simulink model "Thruster_Example_rw"  (R2024b)
settings: Solver=ode4  StartTime=0.0  StopTime=2000  FixedStep=0.01  RelTol=1e-3
undefined symbols (not defined in the file): Cube_L, dt, F_vec, Iws, M_rw, m_tot, norm_Ib, Omega1_init, Omega2_init, Omega3_init, Omega4_init, qb0, rad2rpm, RCS_F, RCS_F_vec, RCS_Pos, RCS_pos, RCS_PWM_Freq, RCS_Sampling_time, RCS_THR_vec, REL_TS_POS_I_0, REL_TS_VEL_I_0, RW_As, RW_Max_Speed, RW_Omegad_max, sat, SC_Ib, SC_state0, SS_Total_Mass, TC_Kepler, THR_dt, THR_Force, THR_freq, THR_Pos, TS_Ib, TS_qb0, TS_state0, TS_wb0, wb0, X, Y, Z
libraries: sm_lib x348, nesl_utility x236, simulink_extras x115, sharedtransform x64, aerolibutil x38, simulink x28, sharedutil x13
(part 15 of 16)

== matlab function Thruster_Example_rw/Reaction_Wheel_Simple1/quaternion to Euler angle 1 ==
  data: angle output; q input
function angle = quat2eulang(q)
% ZYX 회전 가정

% q0 = q(1); q1 = q(2); q2 = q(3); q3 = q(4);
% 
% yaw = atan2(2*(q1*q2 + q0*q3), q0^2+q1^2-q2^2-q3^2);
% 
% s = 2*(q0*q2 - q3*q1);
% s = max(-1, min(1, s));      % clamp
% pitch = asin(s);
% 
% roll = atan2(2*(q2*q3 + q0*q1), q0^2-q1^2-q2^2+q3^2);



% % 'ZYX' 회전에서 DCM을 Body-frame -> 관성좌표계 으로 정의할 때, 각을 구하는 상황.
% % /                cos(psi) cos(theta),                              cos(theta) sin(psi),                   -sin(theta)     \
% % |                                                                                                                         |
% % | cos(psi) sin(phi) sin(theta) - cos(phi) sin(psi), cos(phi) cos(psi) + sin(phi) sin(psi) sin(theta), cos(theta) sin(phi) |
% % |                                                                                                                         |
% % \ sin(phi) sin(psi) + cos(phi) cos(psi) sin(theta), cos(phi) sin(psi) sin(theta) - cos(psi) sin(phi), cos(phi) cos(theta) /
R = quat2DCM(q);
yaw   = atan2(R(1,2), R(1,1));
pitch = -asin(R(1,3));
roll  = atan2(R(2,3), R(3,3));



% angle = [roll, pitch, yaw]';
angle = [yaw, pitch, roll]'; %MATLAB 에서는 [roll, pitch, yaw] 가 아닌 [yaw, pitch, roll] 순으로 값을 반환한다.
% 실제 도움말을 보면, 반환각 벡터에 대해 "Ψ is R1, Θ is R2, and Φ is R3." 으로 나와있는 것을 볼 수 있다.



function R = quat2DCM(q)

q0 = q(1); q1 = q(2); q2 = q(3); q3 = q(4);

%% DCM을 관성좌표계 -> Body-frame 으로 정의할 때의 행렬 
% R = [2*(q0^2 + q1^2)-1, 2*(q1*q2 - q0*q3),2*(q1*q3 + q2*q0);
%      2*(q1*q2 + q0*q3), 2*(q0^2 + q2^2)-1, 2*(q2*q3 - q1*q0);
%      2*(q1*q3 - q2*q0), 2*(q2*q3 + q1*q0), 2*(q0^2 + q3^2)-1];

%% DCM을 Body-frame -> 관성좌표계 으로 정의할 때의 행렬 
R = [q0^2+q1^2-q2^2-q3^2, 2*(q1*q2 + q0*q3), 2*(q1*q3 - q2*q0);
     2*(q1*q2 - q0*q3), q0^2-q1^2+q2^2-q3^2, 2*(q2*q3 + q1*q0);
     2*(q1*q3 + q2*q0), 2*(q2*q3 - q1*q0), q0^2-q1^2-q2^2+q3^2];

end

end

== matlab function Thruster_Example_rw/Prac1/RCS_Position&Attitude_Controller ==
  settings: updateMethod=DISCRETE
  data: r_rel input; v_rel input; r_ref input; v_ref input; a_ref input; q input; q_err input; w_err input; wb input; F_cmd_B output; tau_cmd_B output; m_sc input; Ib input; Kp_pos input; Kd_pos input; Kp_att input; Kd_att input; r_err output; v_err output; q output; q_err_vec output; w_err output; a_cmd output
function [F_cmd_B, tau_cmd_B, r_err, v_err, q, q_err_vec, w_err, a_cmd] = ...
    relative_position_los_controller( ...
    r_rel, v_rel, ...          % [3x1] relative position/velocity
    r_ref, v_ref, a_ref, ...   % [3x1] desired relative pos/vel/acc
    q, q_err, w_err, wb, m_sc, Ib, Kp_pos, Kd_pos, Kp_att, Kd_att)
%#codegen
%
% q, q_los_ref : scalar-first quaternion [qw qx qy qz]'
%                body -> reference
% r_rel, r_ref, v_rel, v_ref, a_ref : reference frame 기준
%
% 출력:
% F_cmd_B   : [3x1] body frame force command
% tau_cmd_B : [3x1] body frame torque command

F_cmd_B   = zeros(3,1);
tau_cmd_B = zeros(3,1);
r_err     = zeros(3,1);
v_err     = zeros(3,1);
q_err_vec = zeros(3,1);
% w_err     = zeros(3,1);
a_cmd     = zeros(3,1);

%% 1) Relative position controller
r_err = r_ref - r_rel;
v_err = v_ref - v_rel;

a_cmd = a_ref + Kp_pos * r_err + Kd_pos * v_err;
F_cmd_R = m_sc * a_cmd;

%% 2) Reference frame -> body frame
% q : body -> reference
% therefore F_B = C_BR' * F_R
C_BR   = quat_to_dcm_sf(q);
F_cmd_B = C_BR' * F_cmd_R;

%% 3) LOS attitude controller

% shortest path
% if q_err(1) < 0
%     q_err = -q_err;
% end

q_err_vec = q_err(2:4);

tau_cmd_B = Kp_att * q_err_vec + Kd_att * w_err + cross(wb, Ib*wb);
end


function q_out = quat_mul_sf(a, b)
% scalar-first quaternion multiplication
q_out = [ a(1)*b(1) - a(2)*b(2) - a(3)*b(3) - a(4)*b(4);
    a(1)*b(2) + a(2)*b(1) + a(3)*b(4) - a(4)*b(3);
    a(1)*b(3) - a(2)*b(4) + a(3)*b(1) + a(4)*b(2);
    a(1)*b(4) + a(2)*b(3) - a(3)*b(2) + a(4)*b(1) ];
end


function C = quat_to_dcm_sf(q)
% scalar-first quaternion, body -> reference
q = q / (sqrt(sum(q.^2)) + 1e-12);

qw = q(1);
qx = q(2);
qy = q(3);
qz = q(4);

C = [1-2*(qy*qy+qz*qz),   2*(qx*qy-qw*qz),   2*(qx*qz+qw*qy);
    2*(qx*qy+qw*qz),     1-2*(qx*qx+qz*qz), 2*(qy*qz-qw*qx);
    2*(qx*qz-qw*qy),     2*(qy*qz+qw*qx),   1-2*(qx*qx+qy*qy)];
end

== matlab function Thruster_Example_rw/Reaction_Wheel_Simple1/deriviation of quaternion1 ==
  data: w input; q_prime output; q input
function q_prime = fcn(w,q)

F_q = (1/2)*[0 -w(1) -w(2) -w(3);
       w(1) 0 w(3) -w(2);
       w(2) -w(3) 0 w(1);
       w(3) w(2) -w(1) 0];

q_prime = F_q*q;

== matlab function Thruster_Example_rw/Prac1/RCS_Relative_Position_Control_Allocation2 ==
  settings: updateMethod=DISCRETE
  data: F_cmd input; tau_cmd input; RCS_pos input; RCS_F_vec input; Tmax input; duty output; F_est output; tau_est output; F_err output; tau_err output; sat_ratio output; wF input; wT input
function [duty, F_est, tau_est, F_err, tau_err, sat_ratio] = ...
    rcs_force_torque_allocator(F_cmd, tau_cmd, RCS_pos, RCS_F_vec, Tmax, wF, wT)
%#codegen
%
% F_cmd      : [3x1] commanded force in body frame [N]
% tau_cmd    : [3x1] commanded torque in body frame [N*m]
% RCS_pos    : [3xN] thruster positions in body frame [m]
% RCS_F_vec  : [3xN] thruster direction vectors
% Tmax       : scalar, max thrust of one thruster [N]
% wF         : scalar, force tracking weight
% wT         : scalar, torque tracking weight
%
% duty       : [N x 1], 0~1
% F_est      : [3x1], achieved force [N]
% tau_est    : [3x1], achieved torque [N*m]
% F_err      : [3x1], force error [N]
% tau_err    : [3x1], torque error [N*m]
% sat_ratio  : saturated thruster ratio

    N = size(RCS_pos, 2);

    duty      = zeros(N,1);
    F_est     = zeros(3,1);
    tau_est   = zeros(3,1);
    F_err     = zeros(3,1);
    tau_err   = zeros(3,1);
    sat_ratio = 0;

    Fmat = zeros(3, N);
    Tmat = zeros(3, N);

    for i = 1:N
        dir_i = RCS_F_vec(:,i);
        nrm   = sqrt(sum(dir_i.^2));

        if nrm > 1e-12
            dir_i = dir_i / nrm;
        else
            dir_i = [0;0;0];
        end

        Fi = Tmax * dir_i;
        Ti = cross3(RCS_pos(:,i), Fi);

        Fmat(:,i) = Fi;
        Tmat(:,i) = Ti;
    end

    % Solve:
    % min || wF*(Fmat*u - F_cmd) ||^2 + || wT*(Tmat*u - tau_cmd) ||^2
    % s.t. 0 <= u <= 1

    A = [wF * Fmat;
         wT * Tmat];

    b = [wF * F_cmd;
         wT * tau_cmd];

    H = A' * A + 1e-8 * eye(N);
    g = A' * b;

    alpha = 1.0 / (trace(H) + 1e-9);
    u = zeros(N,1);

    for k = 1:150
        grad = H * u - g;
        u    = u - alpha * grad;

        for j = 1:N
            if u(j) < 0
                u(j) = 0;
            elseif u(j) > 1
                u(j) = 1;
            end
        end
    end

    duty    = u;
    F_est   = Fmat * duty;
    tau_est = Tmat * duty;

    F_err   = F_cmd   - F_est;
    tau_err = tau_cmd - tau_est;

    sat_ratio = sum(duty > 0.999) / N;
end


function c = cross3(a, b)
    c = [ a(2)*b(3) - a(3)*b(2);
          a(3)*b(1) - a(1)*b(3);
          a(1)*b(2) - a(2)*b(1) ];
end

== matlab function Thruster_Example_rw/Reaction_Wheel_3axis/deriviation of quaternion2 ==
  data: w input; q_prime output; q input
function q_prime = fcn(w,q)

F_q = (1/2)*[0 -w(1) -w(2) -w(3);
       w(1) 0 w(3) -w(2);
       w(2) -w(3) 0 w(1);
       w(3) w(2) -w(1) 0];

q_prime = F_q*q;

== matlab function Thruster_Example_rw/Prac1/SC 6-DOF Dynamics ==
  data: w input; x input; Ib input; m_tot input; Iws input; As input; Omega input; Omegad input; RCS_mea input; RCS_pos input; RCS_vec input; wd output; R_Ib input; T_ext input; F_ext input; xd output
function [wd, xd]  = eq_propagate(w, x, Ib, m_tot, ...
                                   Iws, As, Omega, Omegad, ...
                                   RCS_mea, RCS_pos, RCS_vec, R_Ib, ...
                                   T_ext, F_ext)
% % 
% 출력 1: 위성 동체 좌표계 각가속도
% 출력 2: 관성좌표계 선가속도

RW_h = As*Iws*Omega;
RW_hd = As*Iws*Omegad;
% 
% % % 
% N = 16;
% RCS_f = zeros(3,N);
% RCS_t = zeros(3,N);
% 
% for i = 1:N
%     r_i = RCS_pos(:,i);   % position of thruster i
%     d_i = RCS_vec(:,i);   % thrust direction of thruster i
% 
%     % force contribution
%     RCS_f(:,i) = d_i;
% 
%     % torque contribution
%     RCS_t(:,i) = cross(r_i, d_i);
% end
% RCS_f_total = RCS_f * RCS_mea;  % [3x1]
% RCS_t_total = RCS_t * RCS_mea;  % [3x1]


%% Rotational Motion
wd = [0 0 0]';
wd = inv(Ib)*(T_ext - RW_hd - cross(w, Ib*w + RW_h));

%% Translational Motion

% F_I = R_Ib * RCS_f_total;
F_I = [0 0 0]';

u  = 3.9860064e+14; % earth gravitional parameter
Re = 6378137;      % earth radius [m]

xd = zeros(size(x));

v1_i = x(4); % x1 = dx/dt
v2_i = x(5); % y1 = dy/dt
v3_i = x(6); % z1 = dz/dt
p1_i = x(1); % x
p2_i = x(2); % y
p3_i = x(3); % z

r=sqrt(p1_i^2+p2_i^2+p3_i^2);

% % %   Keplar Motion Equatnion
% % %  => r_dd + u/(r^3)r_ = 0 => r_dd = -u/(r^3)r_
xd(1) = v1_i;
xd(2) = v2_i;
xd(3) = v3_i;
xd(4) = -u*p1_i/(r^3) + F_I(1)/m_tot + F_ext(1)/m_tot;
xd(5) = -u*p2_i/(r^3) + F_I(2)/m_tot + F_ext(2)/m_tot;
xd(6) = -u*p3_i/(r^3) + F_I(3)/m_tot + F_ext(3)/m_tot;

end

== matlab function Thruster_Example_rw/Reaction_Wheel_3axis/quaternion to Euler angle 1 ==
  data: angle output; q input
function angle = quat2eulang(q)
% ZYX 회전 가정

% q0 = q(1); q1 = q(2); q2 = q(3); q3 = q(4);
% 
% yaw = atan2(2*(q1*q2 + q0*q3), q0^2+q1^2-q2^2-q3^2);
% 
% s = 2*(q0*q2 - q3*q1);
% s = max(-1, min(1, s));      % clamp
% pitch = asin(s);
% 
% roll = atan2(2*(q2*q3 + q0*q1), q0^2-q1^2-q2^2+q3^2);



% % 'ZYX' 회전에서 DCM을 Body-frame -> 관성좌표계 으로 정의할 때, 각을 구하는 상황.
% % /                cos(psi) cos(theta),                              cos(theta) sin(psi),                   -sin(theta)     \
% % |                                                                                                                         |
% % | cos(psi) sin(phi) sin(theta) - cos(phi) sin(psi), cos(phi) cos(psi) + sin(phi) sin(psi) sin(theta), cos(theta) sin(phi) |
% % |                                                                                                                         |
% % \ sin(phi) sin(psi) + cos(phi) cos(psi) sin(theta), cos(phi) sin(psi) sin(theta) - cos(psi) sin(phi), cos(phi) cos(theta) /
R = quat2DCM(q);
yaw   = atan2(R(1,2), R(1,1));
pitch = -asin(R(1,3));
roll  = atan2(R(2,3), R(3,3));



% angle = [roll, pitch, yaw]';
angle = [yaw, pitch, roll]'; %MATLAB 에서는 [roll, pitch, yaw] 가 아닌 [yaw, pitch, roll] 순으로 값을 반환한다.
% 실제 도움말을 보면, 반환각 벡터에 대해 "Ψ is R1, Θ is R2, and Φ is R3." 으로 나와있는 것을 볼 수 있다.



function R = quat2DCM(q)

q0 = q(1); q1 = q(2); q2 = q(3); q3 = q(4);

%% DCM을 관성좌표계 -> Body-frame 으로 정의할 때의 행렬 
% R = [2*(q0^2 + q1^2)-1, 2*(q1*q2 - q0*q3),2*(q1*q3 + q2*q0);
%      2*(q1*q2 + q0*q3), 2*(q0^2 + q2^2)-1, 2*(q2*q3 - q1*q0);
%      2*(q1*q3 - q2*q0), 2*(q2*q3 + q1*q0), 2*(q0^2 + q3^2)-1];

%% DCM을 Body-frame -> 관성좌표계 으로 정의할 때의 행렬 
R = [q0^2+q1^2-q2^2-q3^2, 2*(q1*q2 + q0*q3), 2*(q1*q3 - q2*q0);
     2*(q1*q2 - q0*q3), q0^2-q1^2+q2^2-q3^2, 2*(q2*q3 + q1*q0);
     2*(q1*q3 + q2*q0), 2*(q2*q3 - q1*q0), q0^2-q1^2-q2^2+q3^2];

end

end

== matlab function Thruster_Example_rw/Reaction_Wheel_Simple3/deriviation of quaternion2 ==
  data: w input; q_prime output; q input
function q_prime = fcn(w,q)

F_q = (1/2)*[0 -w(1) -w(2) -w(3);
       w(1) 0 w(3) -w(2);
       w(2) -w(3) 0 w(1);
       w(3) w(2) -w(1) 0];

q_prime = F_q*q;

== matlab function Thruster_Example_rw/Reaction_Wheel_Simple3/rigid body2 ==
  data: Wheel_MOI input; Ib input; t_ext input; omega_prime output; omega input; omega_rw input; omega_rw_prime input
function omega_prime = fcn(Wheel_MOI, Ib, t_ext, omega,omega_rw,omega_rw_prime)
% L = [0.3 0.3 0.3]'; %Length([m]) of cube 
% M = 10; %Mass([kg]) of cube
% MOI([kg*m^2]) of cube
% I = [ 1/12*M*(L(2)^2+L(3)^2) 0 0;
%       0 1/12*M*(L(1)^2+L(3)^2) 0;
%       0 0 1/12*M*(L(1)^2+L(2)^2)];

% R=0.015; % Radius([m]) of cylinder(Reaction wheel)
% M_rw=0.01; % Mass([kg]) of cylinder(Reaction wheel)
% L_rw=0.01; % Length([m]) of cylinder(Reaction wheel)

% MOI([kg*m^2]) of cylinder(Reaction wheel)
% I_rw=[1/4*M_rw*R^2+1/12*M_rw*L_rw^2 0 0;
%     0 1/4*M_rw*R^2+1/12*M_rw*L_rw^2 0;
%     0 0 1/2*M_rw*R^2];
% Ib=I;

I_rw3 = Wheel_MOI(3,3);
I_rw = diag([0 0 I_rw3]);

As1 = [0 0 0]';
As2 = [0 0 0]';
As3 = [0 -sind(45) cosd(45)]';

As = [As1, As2, As3];

omega_prime = inv(Ib)*(t_ext - As*I_rw*omega_rw_prime - cross(omega, (Ib*omega) + As*I_rw*omega_rw));

end

== matlab function Thruster_Example_rw/Reaction_Wheel_3axis/rigid body2 ==
  data: Ib input; t_ext input; omega_prime output; omega input; omega_rw input; omega_rw_prime input; R_rw input; L_rw input; M_rw input
function omega_prime = fcn(Ib, t_ext, omega,omega_rw,omega_rw_prime, R_rw, L_rw, M_rw)
L = [0.3 0.3 0.3]'; %Length([m]) of cube 
M = 10; %Mass([kg]) of cube
% MOI([kg*m^2]) of cube
I = [ 1/12*M*(L(2)^2+L(3)^2) 0 0;
      0 1/12*M*(L(1)^2+L(3)^2) 0;
      0 0 1/12*M*(L(1)^2+L(2)^2)];

% R=0.015; % Radius([m]) of cylinder(Reaction wheel)
% L_rw=0.01; % Length([m]) of cylinder(Reaction wheel)
% M_rw=0.01; % Mass([kg]) of cylinder(Reaction wheel)
R=R_rw;


% MOI([kg*m^2]) of cylinder(Reaction wheel)
I_rw=[1/4*M_rw*R^2+1/12*M_rw*L_rw^2 0 0;
    0 1/4*M_rw*R^2+1/12*M_rw*L_rw^2 0;
    0 0 1/2*M_rw*R^2];

% Ib=I;


omega_prime = inv(Ib)*(t_ext - I_rw*omega_rw_prime - cross(omega, (Ib*omega) + I_rw*omega_rw));

end

== matlab function Thruster_Example_rw/Reaction_Wheel_Simple2/deriviation of quaternion2 ==
  data: w input; q_prime output; q input
function q_prime = fcn(w,q)

F_q = (1/2)*[0 -w(1) -w(2) -w(3);
       w(1) 0 w(3) -w(2);
       w(2) -w(3) 0 w(1);
       w(3) w(2) -w(1) 0];

q_prime = F_q*q;

== matlab function Thruster_Example_rw/Single_Reaction_Wheel_PD_Control/deriviation of quaternion2 ==
  data: w input; q_prime output; q input
function q_prime = fcn(w,q)

F_q = (1/2)*[0 -w(1) -w(2) -w(3);
       w(1) 0 w(3) -w(2);
       w(2) -w(3) 0 w(1);
       w(3) w(2) -w(1) 0];

q_prime = F_q*q;

== matlab function Thruster_Example_rw/Single_Reaction_Wheel_PD_Control/rigid body2 ==
  data: Wheel_MOI input; Ib input; t_ext input; omega_prime output; omega input; omega_rw input; omega_rw_prime input
function omega_prime = fcn(Wheel_MOI, Ib, t_ext, omega,omega_rw,omega_rw_prime)
% L = [0.3 0.3 0.3]'; %Length([m]) of cube 
% M = 10; %Mass([kg]) of cube
% MOI([kg*m^2]) of cube
% I = [ 1/12*M*(L(2)^2+L(3)^2) 0 0;
%       0 1/12*M*(L(1)^2+L(3)^2) 0;
%       0 0 1/12*M*(L(1)^2+L(2)^2)];

% R=0.015; % Radius([m]) of cylinder(Reaction wheel)
% M_rw=0.01; % Mass([kg]) of cylinder(Reaction wheel)
% L_rw=0.01; % Length([m]) of cylinder(Reaction wheel)

% MOI([kg*m^2]) of cylinder(Reaction wheel)
% I_rw=[1/4*M_rw*R^2+1/12*M_rw*L_rw^2 0 0;
%     0 1/4*M_rw*R^2+1/12*M_rw*L_rw^2 0;
%     0 0 1/2*M_rw*R^2];
% Ib=I;

I_rw3 = Wheel_MOI(3,3);
I_rw = diag([0 0 I_rw3]);

As1 = [0 0 0]';
As2 = [0 0 0]';
As3 = [0 -sind(45) cosd(45)]';

As = [As1, As2, As3];

omega_prime = inv(Ib)*(t_ext - As*I_rw*omega_rw_prime - cross(omega, (Ib*omega) + As*I_rw*omega_rw));

end

== matlab function Thruster_Example_rw/Single_Reaction_Wheel_PD_Control/rigid body1 ==
  data: yaw_err input; w_z_err input; u_cntl output
function u_cntl = fcn(yaw_err, w_z_err)

K1 = 0.0;
K2 = 100000.0;

u_cntl = K1*yaw_err + K2*w_z_err;


end

== matlab function Thruster_Example_rw/Reaction_Wheel_another_Position/deriviation of quaternion2 ==
  data: w input; q_prime output; q input
function q_prime = fcn(w,q)

F_q = (1/2)*[0 -w(1) -w(2) -w(3);
       w(1) 0 w(3) -w(2);
       w(2) -w(3) 0 w(1);
       w(3) w(2) -w(1) 0];

q_prime = F_q*q;

== matlab function Thruster_Example_rw/Reaction_Wheel_Simple2/rigid body2 ==
  data: Wheel_MOI input; Ib input; t_ext input; omega_prime output; omega input; omega_rw input; omega_rw_prime input
function omega_prime = fcn(Wheel_MOI, Ib, t_ext, omega,omega_rw,omega_rw_prime)
% L = [0.3 0.3 0.3]'; %Length([m]) of cube 
% M = 10; %Mass([kg]) of cube
% MOI([kg*m^2]) of cube
% I = [ 1/12*M*(L(2)^2+L(3)^2) 0 0;
%       0 1/12*M*(L(1)^2+L(3)^2) 0;
%       0 0 1/12*M*(L(1)^2+L(2)^2)];

% R=0.015; % Radius([m]) of cylinder(Reaction wheel)
% M_rw=0.01; % Mass([kg]) of cylinder(Reaction wheel)
% L_rw=0.01; % Length([m]) of cylinder(Reaction wheel)

% MOI([kg*m^2]) of cylinder(Reaction wheel)
% I_rw=[1/4*M_rw*R^2+1/12*M_rw*L_rw^2 0 0;
%     0 1/4*M_rw*R^2+1/12*M_rw*L_rw^2 0;
%     0 0 1/2*M_rw*R^2];
% Ib=I;

I_rw1 = Wheel_MOI(3,3);
I_rw = diag([I_rw1 I_rw1 I_rw1]);

omega_prime = inv(Ib)*(t_ext - I_rw*omega_rw_prime - cross(omega, (Ib*omega) + I_rw*omega_rw));

end

== matlab function Thruster_Example_rw/Reaction_Wheel_another_Position/rigid body2 ==
  data: Wheel_MOI input; Ib input; t_ext input; omega_prime output; omega input; omega_rw input; omega_rw_prime input
function omega_prime = fcn(Wheel_MOI, Ib, t_ext, omega,omega_rw,omega_rw_prime)

% Ib = diag([0.15, 0.15, 0.15]);
I_rw3 = Wheel_MOI(3,3);
% I_rw3 = 0.001125;

I_rw = diag([0 0 I_rw3]);

As1 = [0 0 0]';
As2 = [0 0 0]';
% As3 = [0 -sind(45) cosd(45)]';
As3 = [0 0 1]';

As = [As1, As2, As3];

omega_prime = inv(Ib)*(t_ext - As*I_rw*omega_rw_prime - cross(omega, (Ib*omega) + As*I_rw*omega_rw));

end

== matlab function Thruster_Example_rw/Reaction_Wheel_3axis(with 4 wheels)/deriviation of quaternion2 ==
  data: w input; q_prime output; q input
function q_prime = fcn(w,q)

F_q = (1/2)*[0 -w(1) -w(2) -w(3);
       w(1) 0 w(3) -w(2);
       w(2) -w(3) 0 w(1);
       w(3) w(2) -w(1) 0];

q_prime = F_q*q;

== matlab function Thruster_Example_rw/Reaction_Wheel_3axis(with 4 wheels)/rigid body2 ==
  data: Wheel_MOI input; Ib input; t_ext input; omega_prime output; omega input; omega_rw input; omega_rw_prime input
function omega_prime = fcn(Wheel_MOI, Ib, t_ext, omega,omega_rw,omega_rw_prime)
% L = [0.3 0.3 0.3]'; %Length([m]) of cube 
% M = 10; %Mass([kg]) of cube
% % MOI([kg*m^2]) of cube
% I = [ 1/12*M*(L(2)^2+L(3)^2) 0 0;
%       0 1/12*M*(L(1)^2+L(3)^2) 0;
%       0 0 1/12*M*(L(1)^2+L(2)^2)];

% R=0.015; % Radius([m]) of cylinder(Reaction wheel)
% M_rw=0.01; % Mass([kg]) of cylinder(Reaction wheel)
% L_rw=0.01; % Length([m]) of cylinder(Reaction wheel)

% MOI([kg*m^2]) of cylinder(Reaction wheel)
% I_rw=[1/4*M_rw*R^2+1/12*M_rw*L_rw^2 0 0;
%     0 1/4*M_rw*R^2+1/12*M_rw*L_rw^2 0;
%     0 0 1/2*M_rw*R^2];
% Ib=I;

I_rw1 = Wheel_MOI(3,3);
I_rw = diag([I_rw1 I_rw1 I_rw1]);

omega_prime = inv(Ib)*(t_ext - I_rw*omega_rw_prime - cross(omega, (Ib*omega) + I_rw*omega_rw));

end

== matlab function Thruster_Example_rw/Prac1/Subsystem/Attitude_PD_control ==
  settings: updateMethod=DISCRETE
  data: u_torq output; q_err input; w_err input
function u_torq = att_pd_control(q_err, w_err)

persistent first_flg
persistent I_save

dt = 0.01;

if isempty(first_flg)
    first_flg = 1;
    I_save = [0 0 0]';
end

K1 = 10.1*diag([1 1 1]);
K2 = 8.2*diag([1 1 1]);
K3 = 0.1*diag([1 1 1]);

q_err_ = [q_err(2), q_err(3), q_err(4)]';

u_torq = K1*q_err_ + K2*w_err + K3*I_save;

I_save = I_save + q_err_ * dt;

end

== matlab function Thruster_Example_rw/Prac1/Subsystem/Attitude_PD_control1 ==
  settings: updateMethod=DISCRETE
  data: F_B_cmd output; r_I input; v_I input; q_IB input; r_d input; v_d input; a_d input; m input
function F_B_cmd  = CTRL_WRENCH_6DOF(r_I, v_I, q_IB, r_d, v_d, a_d, m)
%#codegen
% ============================================================
% Controller block
% Input :
%   r_I      [3x1] current position in inertial frame
%   v_I      [3x1] current velocity in inertial frame
%   q_IB     [4x1] quaternion [qw qx qy qz], Body -> Inertial
%   omega_B  [3x1] current angular velocity in body frame
%
%   r_d      [3x1] desired position in inertial frame
%   v_d      [3x1] desired velocity in inertial frame
%   a_d      [3x1] desired acceleration in inertial frame
%   q_d      [4x1] desired quaternion, Body -> Inertial
%   omega_d_B[3x1] desired angular velocity in body frame
%
%   m        scalar mass
%   J        [3x3] inertia matrix in body frame
%
% Output:
%   F_B_cmd    [3x1] desired total body force
%   tau_B_cmd  [3x1] desired total body torque
% ============================================================

    % -------------------------
    % Quaternion normalize
    % -------------------------
    q_IB = quat_normalize(q_IB); 

    % -------------------------
    % Gains (example)
    % -------------------------
    Kp_r = 10*diag([0.01, 0.006, 0.006]);   % position gain
    Kd_r = 100*diag([0.01, 0.01, 0.01]);   % velocity damping
 
    % Kp_r = diag([0.010, 0.010, 0.010]);   % position gain
    % Kd_r = diag([0.060, 0.060, 0.060]);   % velocity damping

    % -------------------------
    % Position control
    % inertial acceleration command
    % -------------------------
    e_r = r_I - r_d;
    e_v = v_I - v_d;

    a_cmd   = a_d - Kp_r * e_r - Kd_r * e_v;
    F_I_cmd = m * a_cmd;

    % Convert inertial force -> body force
    R_IB    = quat_to_rotm(q_IB);
    F_B_cmd = R_IB.' * F_I_cmd;
 
end


% ============================================================
% Local helper functions
% ============================================================

function qn = quat_normalize(q)
    n = norm(q);
    if n < 1e-12
        qn = [1;0;0;0];
    else
        qn = q / n;
    end
end
 

function R = quat_to_rotm(q)
    % q = [qw qx qy qz], Body -> Inertial
    qw = q(1); qx = q(2); qy = q(3); qz = q(4);

    R = [1-2*(qy^2+qz^2),   2*(qx*qy-qz*qw),   2*(qx*qz+qy*qw);
         2*(qx*qy+qz*qw),   1-2*(qx^2+qz^2),   2*(qy*qz-qx*qw);
         2*(qx*qz-qy*qw),   2*(qy*qz+qx*qw),   1-2*(qx^2+qy^2)];
end

== matlab function Thruster_Example_rw/Thruster_Example_1/Attitude_PD_control ==
  settings: updateMethod=DISCRETE
  data: u_torq output; q_err input; w_err input
function u_torq = att_pd_control(q_err, w_err)

persistent first_flg
persistent I_save

dt = 0.01;

if isempty(first_flg)
    first_flg = 1;
    I_save = [0 0 0]';
end

K1 = 0.2*diag([1 1 1]);
K2 = 0.4*diag([1 1 1]);
K3 = 0.02*diag([1 1 1]);

q_err_ = [q_err(2), q_err(3), q_err(4)]';

u_torq = K1*q_err_ + K2*w_err + K3*I_save;

I_save = I_save + q_err_ * dt;

end

== matlab function Thruster_Example_rw/Thruster_Example_1/Rigid_Body ==
  data: t_ext input; wd output; w input; F_pwm_mea input; F_vec input; r_thr input
function wd = fcn(t_ext, w, F_pwm_mea, F_vec, r_thr)

Ib = diag([0.015, 0.015, 0.015]);

t_thr = [0 0 0]';
for i=1:12
    Fi = F_pwm_mea(i).*F_vec(:,i);
    Ti = cross(Fi, r_thr(:,i));
    t_thr = t_thr + Ti;
end

wd = inv(Ib)*(t_ext + t_thr - cross(w,Ib*w));

end

== matlab function Thruster_Example_rw/Prac2/deriviation of quaternion1 ==
  data: w input; q_prime output; q input
function q_prime = fcn(w,q)

F_q = (1/2)*[0 -w(1) -w(2) -w(3);
       w(1) 0 w(3) -w(2);
       w(2) -w(3) 0 w(1);
       w(3) w(2) -w(1) 0];

q_prime = F_q*q;

== matlab function Thruster_Example_rw/Thruster_Example_1/Triggered Subsystem/Rigid_Body1 ==
  data: tau_cmd input; THR_Pos input; F_vec input; u_pwm output; Ts input; t_on output; tau_ach_row output; f_ach_row output; cost output
function [u_pwm, t_on, tau_ach_row, f_ach_row, cost] = RCS_AttitudePWM_QP(tau_cmd, THR_Pos, F_vec, Ts)
%#codegen
% ============================================================
% 12-thruster RCS attitude PWM allocation via box-QP
% Decision variable: u_pwm in [0,1] (PWM duty)
%
% Average model:
%   f_avg   = A_f   * u
%   tau_avg = A_tau * u
%
% Cost:
%   0.5||A_tau u - tau_cmd||^2_{W} + 0.5*gamma||A_f u||^2
%   + 0.5*lambda||u-u_prev||^2 + rho*sum(u)
% s.t. 0 <= u <= 1
%
% Outputs:
%   u_pwm       [12x1]
%   t_on        [12x1]
%   tau_ach_row [1x3]  (to avoid 3x1 matrix dimension mismatch)
%   f_ach_row   [1x3]
%   cost        [1x1]
% ============================================================

% ---------- USER: fill these for your thruster geometry ----------
persistent r_b d_b F_on
persistent Wtau gamma lambda rho
persistent Niter powerIters
persistent u_prev

if isempty(r_b)
    % === TODO: replace with your real layout ===
    % r_b = zeros(3,12);        % [m] CoM -> thruster location (body frame)
    % d_b = zeros(3,12);        % [-] thrust direction unit vectors (body frame)
    r_b = THR_Pos;        % [m] CoM -> thruster location (body frame)
    d_b = F_vec;        % [-] thrust direction unit vectors (body frame)

    F_on = 0.01*ones(1,12);        % [N] thrust when ON

    % Weights (tune)
    Wtau   = 10*eye(3);
    gamma  = 0.5;             % net force penalty
    lambda = 0.005;            % smoothness penalty
    rho    = 0.0001;             % fuel proxy

    % Solver iterations
    Niter      = 50;
    powerIters = 10;

    u_prev = zeros(12,1);
end

% ---------- Build A_f and A_tau ----------
A_f   = zeros(3,12);
A_tau = zeros(3,12);

for i = 1:12
    fi = F_on(i) * d_b(:,i);     % 3x1
    A_f(:,i) = fi;

    r = r_b(:,i);
    % cross(r, fi)
    A_tau(1,i) = r(2)*fi(3) - r(3)*fi(2);
    A_tau(2,i) = r(3)*fi(1) - r(1)*fi(3);
    A_tau(3,i) = r(1)*fi(2) - r(2)*fi(1);
end

% ---------- QP in quadratic form ----------
H = (A_tau' * Wtau * A_tau) + gamma*(A_f' * A_f) + lambda*eye(12);
f = -(A_tau' * Wtau * tau_cmd) - lambda*u_prev + rho*ones(12,1);

% ---------- Projected gradient (codegen-friendly) ----------
u = u_prev;

% Lipschitz estimate via power iteration
v = ones(12,1);
v = v / sqrt(v'*v + 1e-12);
for k = 1:powerIters
    v = H * v;
    nv = sqrt(v'*v + 1e-12);
    v = v / nv;
end
L = v' * (H * v);
alpha = 1.0 / (L + 1e-6);

for k = 1:Niter
    g = H*u + f;
    u = u - alpha*g;

    % projection to [0,1]
    for i = 1:12
        if u(i) < 0.0
            u(i) = 0.0;
        elseif u(i) > 1.0
            u(i) = 1.0;
        end
    end
end

u_pwm = u;
t_on  = u_pwm * Ts;

% achieved average force/torque
tau_ach = A_tau * u_pwm;   % 3x1
f_ach   = A_f   * u_pwm;   % 3x1

% output as 1x3 row vectors to avoid [3x1] matrix signal mismatch
tau_ach_row = tau_ach.';   % 1x3
f_ach_row   = f_ach.';     % 1x3

% cost (use previous u_prev BEFORE update)
e_tau = (A_tau*u_pwm - tau_cmd);
cost = 0.5*(e_tau.'*Wtau*e_tau) ...
       + 0.5*gamma*(f_ach.'*f_ach) ...
       + 0.5*lambda*((u_pwm-u_prev).'* (u_pwm-u_prev)) ...
       + rho*sum(u_pwm);

% warm start update
u_prev = u_pwm;

end

== matlab function Thruster_Example_rw/Thruster_Example_1/THR_Allocation ==
  data: pwm output; tau_cmd input; F_on input; f input; r_thr input
function pwm = RCS_Torque2PWM(tau_cmd, F_on, f, r_thr)
%#codegen
% ============================================================
% Minimal RCS allocation: torque command -> PWM duty (0..1)
%   tau ≈ sum_i r_i x (f_i * F_on_i * pwm_i)
%
% Inputs:
%   tau_cmd [3x1]
%   F_on    scalar or [12x1]
%   f       [3x12]  (columns are unit vectors)
%   r_thr   [3x12]  (columns are position vectors wrt CoM)
%
% Output:
%   pwm     [12x1] duty in [0,1]
% ============================================================

% F_on -> 12x1
if isscalar(F_on)
    Fon = F_on * ones(12,1);
else
    Fon = F_on(:);
end

% Build effectiveness matrix B (3x12): tau = B * pwm
B = zeros(3,12);
for i = 1:12
    Fi = Fon(i);
    B(:,i) = cross3(r_thr(:,i), f(:,i) * Fi);  % torque from pwm=1
end

% Unconstrained least-squares solution (minimum-norm)
pwm = B' * ((B*B') \ tau_cmd);

% Clamp to [0,1]
for i=1:12
    if pwm(i) < 0, pwm(i) = 0; end
    if pwm(i) > 1, pwm(i) = 1; end
end

end

function c = cross3(a,b)
c = [ a(2)*b(3) - a(3)*b(2);
      a(3)*b(1) - a(1)*b(3);
      a(1)*b(2) - a(2)*b(1) ];
end

== matlab function Thruster_Example_rw/Thruster_Example_1/Quaternion_Kinematics ==
  data: w input; qd output; q input
function qd = fcn(w,q)

F_q = (1/2)*[0 -w(1) -w(2) -w(3);
       w(1) 0 w(3) -w(2);
       w(2) -w(3) 0 w(1);
       w(3) w(2) -w(1) 0];

qd = F_q*q;

end

== matlab function Thruster_Example_rw/Prac2/deriviation of quaternion2 ==
  data: w input; q_prime output; q input
function q_prime = fcn(w,q)

F_q = (1/2)*[0 -w(1) -w(2) -w(3);
       w(1) 0 w(3) -w(2);
       w(2) -w(3) 0 w(1);
       w(3) w(2) -w(1) 0];

q_prime = F_q*q;

== matlab function Thruster_Example_rw/Prac2/diff_angle ==
  data: angle_err output; q_err input
function angle_err = calc_diff(q_err)

% normalize
q_err = q_err / norm(q_err);

% safe scalar part
q0 = min(abs(q_err(1)),1);

% angle
angle_err = 2*acos(q0);

end

== matlab function Thruster_Example_rw/Prac2/quaternion to Euler angle 1 ==
  data: angle output; q input
function angle = quat2eulang(q)
% ZYX 회전 가정

% q0 = q(1); q1 = q(2); q2 = q(3); q3 = q(4);
% 
% yaw = atan2(2*(q1*q2 + q0*q3), q0^2+q1^2-q2^2-q3^2);
% 
% s = 2*(q0*q2 - q3*q1);
% s = max(-1, min(1, s));      % clamp
% pitch = asin(s);
% 
% roll = atan2(2*(q2*q3 + q0*q1), q0^2-q1^2-q2^2+q3^2);



% % 'ZYX' 회전에서 DCM을 Body-frame -> 관성좌표계 으로 정의할 때, 각을 구하는 상황.
% % /                cos(psi) cos(theta),                              cos(theta) sin(psi),                   -sin(theta)     \
% % |                                                                                                                         |
% % | cos(psi) sin(phi) sin(theta) - cos(phi) sin(psi), cos(phi) cos(psi) + sin(phi) sin(psi) sin(theta), cos(theta) sin(phi) |
% % |                                                                                                                         |
% % \ sin(phi) sin(psi) + cos(phi) cos(psi) sin(theta), cos(phi) sin(psi) sin(theta) - cos(psi) sin(phi), cos(phi) cos(theta) /
R = quat2DCM(q);
yaw   = atan2(R(1,2), R(1,1));
pitch = -asin(R(1,3));
roll  = atan2(R(2,3), R(3,3));



% angle = [roll, pitch, yaw]';
angle = [yaw, pitch, roll]'; %MATLAB 에서는 [roll, pitch, yaw] 가 아닌 [yaw, pitch, roll] 순으로 값을 반환한다.
% 실제 도움말을 보면, 반환각 벡터에 대해 "Ψ is R1, Θ is R2, and Φ is R3." 으로 나와있는 것을 볼 수 있다.



function R = quat2DCM(q)

q0 = q(1); q1 = q(2); q2 = q(3); q3 = q(4);

%% DCM을 관성좌표계 -> Body-frame 으로 정의할 때의 행렬 
% R = [2*(q0^2 + q1^2)-1, 2*(q1*q2 - q0*q3),2*(q1*q3 + q2*q0);
%      2*(q1*q2 + q0*q3), 2*(q0^2 + q2^2)-1, 2*(q2*q3 - q1*q0);
%      2*(q1*q3 - q2*q0), 2*(q2*q3 + q1*q0), 2*(q0^2 + q3^2)-1];

%% DCM을 Body-frame -> 관성좌표계 으로 정의할 때의 행렬 
R = [q0^2+q1^2-q2^2-q3^2, 2*(q1*q2 + q0*q3), 2*(q1*q3 - q2*q0);
     2*(q1*q2 - q0*q3), q0^2-q1^2+q2^2-q3^2, 2*(q2*q3 + q1*q0);
     2*(q1*q3 + q2*q0), 2*(q2*q3 - q1*q0), q0^2-q1^2-q2^2+q3^2];

end

end

== matlab function Thruster_Example_rw/Prac2/rigid body ==
  data: t_ext input; omega_prime output; omega input
function omega_prime = fcn(t_ext, omega)
L = [0.3 0.3 0.3]'; %Length([m]) of cube 
M = 10; %Mass([kg]) of cube

% Density([kg/m^3]) of cube
density = M/(L(1)*L(2)*L(3));   
% MOI([kg*m^2]) of cube
I = [ 1/12*M*(L(2)^2+L(3)^2) 0 0;
      0 1/12*M*(L(1)^2+L(3)^2) 0;
      0 0 1/12*M*(L(1)^2+L(2)^2)];

omega_prime = inv(I)*(t_ext - cross(omega,I*omega));

== matlab function Thruster_Example_rw/Prac2/rigid body1 ==
  data: w input; q_prime output; q input
function q_prime = fcn(w,q)

F_q = (1/2)*[0 -w(1) -w(2) -w(3);
       w(1) 0 w(3) -w(2);
       w(2) -w(3) 0 w(1);
       w(3) w(2) -w(1) 0];

q_prime = F_q*q;

== matlab function Thruster_Example_rw/Prac2/rigid body2 ==
  data: angle output; q input
function angle = quat2eulang(q)
% ZYX 회전 가정

% q0 = q(1); q1 = q(2); q2 = q(3); q3 = q(4);
% 
% yaw = atan2(2*(q1*q2 + q0*q3), q0^2+q1^2-q2^2-q3^2);
% 
% s = 2*(q0*q2 - q3*q1);
% s = max(-1, min(1, s));      % clamp
% pitch = asin(s);
% 
% roll = atan2(2*(q2*q3 + q0*q1), q0^2-q1^2-q2^2+q3^2);



% % 'ZYX' 회전에서 DCM을 Body-frame -> 관성좌표계 으로 정의할 때, 각을 구하는 상황.
% % /                cos(psi) cos(theta),                              cos(theta) sin(psi),                   -sin(theta)     \
% % |                                                                                                                         |
% % | cos(psi) sin(phi) sin(theta) - cos(phi) sin(psi), cos(phi) cos(psi) + sin(phi) sin(psi) sin(theta), cos(theta) sin(phi) |
% % |                                                                                                                         |
% % \ sin(phi) sin(psi) + cos(phi) cos(psi) sin(theta), cos(phi) sin(psi) sin(theta) - cos(psi) sin(phi), cos(phi) cos(theta) /
R = quat2DCM(q);
yaw   = atan2(R(1,2), R(1,1));
pitch = -asin(R(1,3));
roll  = atan2(R(2,3), R(3,3));



% angle = [roll, pitch, yaw]';
angle = [yaw, pitch, roll]'; %MATLAB 에서는 [roll, pitch, yaw] 가 아닌 [yaw, pitch, roll] 순으로 값을 반환한다.
% 실제 도움말을 보면, 반환각 벡터에 대해 "Ψ is R1, Θ is R2, and Φ is R3." 으로 나와있는 것을 볼 수 있다.



function R = quat2DCM(q)

q0 = q(1); q1 = q(2); q2 = q(3); q3 = q(4);

%% DCM을 관성좌표계 -> Body-frame 으로 정의할 때의 행렬 
% R = [2*(q0^2 + q1^2)-1, 2*(q1*q2 - q0*q3),2*(q1*q3 + q2*q0);
%      2*(q1*q2 + q0*q3), 2*(q0^2 + q2^2)-1, 2*(q2*q3 - q1*q0);
%      2*(q1*q3 - q2*q0), 2*(q2*q3 + q1*q0), 2*(q0^2 + q3^2)-1];

%% DCM을 Body-frame -> 관성좌표계 으로 정의할 때의 행렬 
R = [q0^2+q1^2-q2^2-q3^2, 2*(q1*q2 + q0*q3), 2*(q1*q3 - q2*q0);
     2*(q1*q2 - q0*q3), q0^2-q1^2+q2^2-q3^2, 2*(q2*q3 + q1*q0);
     2*(q1*q3 + q2*q0), 2*(q2*q3 - q1*q0), q0^2-q1^2-q2^2+q3^2];

end

end

== matlab function Thruster_Example_rw/Prac2/rigid body3 ==
  data: Ib input; t_ext input; omega_prime output; omega input; omega_rw input; omega_rw_prime input; R_rw input; L_rw input; M_rw input
function omega_prime = fcn(Ib, t_ext, omega,omega_rw,omega_rw_prime, R_rw, L_rw, M_rw)
L = [0.3 0.3 0.3]'; %Length([m]) of cube 
M = 10; %Mass([kg]) of cube
% MOI([kg*m^2]) of cube
I = [ 1/12*M*(L(2)^2+L(3)^2) 0 0;
      0 1/12*M*(L(1)^2+L(3)^2) 0;
      0 0 1/12*M*(L(1)^2+L(2)^2)];

% R=0.015; % Radius([m]) of cylinder(Reaction wheel)
% L_rw=0.01; % Length([m]) of cylinder(Reaction wheel)
% M_rw=0.01; % Mass([kg]) of cylinder(Reaction wheel)
R=R_rw;


% MOI([kg*m^2]) of cylinder(Reaction wheel)
I_rw=[1/4*M_rw*R^2+1/12*M_rw*L_rw^2 0 0;
    0 1/4*M_rw*R^2+1/12*M_rw*L_rw^2 0;
    0 0 1/2*M_rw*R^2];

% Ib=I;


omega_prime = inv(Ib)*(t_ext - I_rw*omega_rw_prime - cross(omega, (Ib*omega) + I_rw*omega_rw));

end

== matlab function Thruster_Example_rw/Prac2/rigid body4 ==
  data: Wheel_MOI input; Ib input; t_ext input; omega_prime output; omega input; omega_rw input; omega_rw_prime input
function omega_prime = fcn(Wheel_MOI, Ib, t_ext, omega,omega_rw,omega_rw_prime)
% L = [0.3 0.3 0.3]'; %Length([m]) of cube 
% M = 10; %Mass([kg]) of cube
% % MOI([kg*m^2]) of cube
% I = [ 1/12*M*(L(2)^2+L(3)^2) 0 0;
%       0 1/12*M*(L(1)^2+L(3)^2) 0;
%       0 0 1/12*M*(L(1)^2+L(2)^2)];

% R=0.015; % Radius([m]) of cylinder(Reaction wheel)
% M_rw=0.01; % Mass([kg]) of cylinder(Reaction wheel)
% L_rw=0.01; % Length([m]) of cylinder(Reaction wheel)

% MOI([kg*m^2]) of cylinder(Reaction wheel)
% I_rw=[1/4*M_rw*R^2+1/12*M_rw*L_rw^2 0 0;
%     0 1/4*M_rw*R^2+1/12*M_rw*L_rw^2 0;
%     0 0 1/2*M_rw*R^2];
% Ib=I;

I_rw1 = Wheel_MOI(3,3);
I_rw = diag([I_rw1 I_rw1 I_rw1]);

omega_prime = inv(Ib)*(t_ext - I_rw*omega_rw_prime - cross(omega, (Ib*omega) + I_rw*omega_rw));

end

== matlab function Thruster_Example_rw/rigid body/rigid body ==
  data: t_ext input; omega_prime output; omega input
function omega_prime = fcn(t_ext, omega)
L = [0.3 0.3 0.3]'; %Length([m]) of cube 
M = 1; %Mass([kg]) of cube

% Density([kg/m^3]) of cube
density = M/(L(1)*L(2)*L(3));   
% MOI([kg*m^2]) of cube
I = [ 1/12*M*(L(2)^2+L(3)^2) 0 0;
      0 1/12*M*(L(1)^2+L(3)^2) 0;
      0 0 1/12*M*(L(1)^2+L(2)^2)];

omega_prime = inv(I)*(t_ext - cross(omega,I*omega));

== matlab function Thruster_Example_rw/Prac1/Subsystem/Attitude_PD_control2 ==
  settings: updateMethod=DISCRETE
  data: q_err input; omega_B input; omega_d_B input; J input; tau_B_cmd output
function tau_B_cmd  = CTRL_WRENCH_6DOF(q_err, omega_B, omega_d_B, J)
%#codegen
% ============================================================
% Controller block
% Input :
%   r_I      [3x1] current position in inertial frame
%   v_I      [3x1] current velocity in inertial frame
%   q_IB     [4x1] quaternion [qw qx qy qz], Body -> Inertial
%   omega_B  [3x1] current angular velocity in body frame
%
%   r_d      [3x1] desired position in inertial frame
%   v_d      [3x1] desired velocity in inertial frame
%   a_d      [3x1] desired acceleration in inertial frame
%   q_d      [4x1] desired quaternion, Body -> Inertial
%   omega_d_B[3x1] desired angular velocity in body frame
%
%   m        scalar mass
%   J        [3x3] inertia matrix in body frame
%
% Output:
%   F_B_cmd    [3x1] desired total body force
%   tau_B_cmd  [3x1] desired total body torque
% ============================================================
 
    % -------------------------
    % Gains (example)
    % -------------------------
    Kq   = J*diag([0.3, 0.3, 0.3]);   % attitude gain
    Kw   = J*diag([5, 5, 5]);   % angular-rate damping

    % Kq   = diag([10.0, 10.0, 10.0]);   % attitude gain
    % Kw   = diag([6.0,  6.0,  6.0 ]);   % angular-rate damping
    % -------------------------
 
    % -------------------------
    % Attitude control 
    % -------------------------
 
    % shortest-path quaternion
    if q_err(1) < 0
        q_err = -q_err;
    end

    e_w = omega_B - omega_d_B;

    % PD + gyro compensation
    tau_B_cmd = -Kq * q_err(2:4) ...
                -Kw * e_w ...
                +cross(omega_B, J * omega_B);
end


% ============================================================
% Local helper functions
% ============================================================

function qn = quat_normalize(q)
    n = norm(q);
    if n < 1e-12
        qn = [1;0;0;0];
    else
        qn = q / n;
    end
end

function qc = quat_conj(q)
    qc = [q(1); -q(2); -q(3); -q(4)];
end

function q = quat_mul(q1, q2)
    % Hamilton product
    w1 = q1(1); x1 = q1(2); y1 = q1(3); z1 = q1(4);
    w2 = q2(1); x2 = q2(2); y2 = q2(3); z2 = q2(4);

    q = [ w1*w2 - x1*x2 - y1*y2 - z1*z2;
          w1*x2 + x1*w2 + y1*z2 - z1*y2;
          w1*y2 - x1*z2 + y1*w2 + z1*x2;
          w1*z2 + x1*y2 - y1*x2 + z1*w2 ];
end

== matlab function Thruster_Example_rw/Prac1/Subsystem/MATLAB Function1 ==
  data: kepel input; statvec output
function statvec  = kepel_statvec (kepel)
%  [statvec] = kepel_statvec (kepel)
%	The function kepel_statvec transforms the keplerian
%	elements kepel into the corresponding state vector in
%	the same reference system.
%
% Input:
%	kepel
% 		vector containing the keplerian elements:
%		(1) - semimajor axis of the orbit in meters.
%		(2) - eccentricity.
%		(3) - inclinatsion in radians.
%		(4) - right ascension of ascending node in radians.
%		(5) - argument of perigee in radians.
%		(6) - mean anomaly in radians.
% Output:
%	statvec
%  		state vector in meters and meters/second.
%
% Authors:
%	Helio K. Kuga;
%	Valder M. Medeiros;
%	Valdemir Carrara		february/80		version 1.0
%	Valdemir Carrara		july 2005		(C version)
%   Valdemir Carrara            March/09        Matlab

EARTH_GRAVITY	= 3.9860064e+14;		% Earth's gravitational constant (m**3/s**2)

a    = kepel(1);	% semi-major axis
exc  = kepel(2);	% eccentricity

c1   = sqrt(1. - exc*exc);

%     rotation matrix

orb2iner = rotmaz(-kepel(4))*rotmax(-kepel(3))*rotmaz(-kepel(5));

%     Kepler's equation

E    = kepler(kepel(6), exc);

sE   = sin(E);
cE   = cos(E);
c3   = sqrt(EARTH_GRAVITY/a)/(1. - exc*cE);

%     state vector

statvec = [[a*(cE - exc), a*c1*sE, 0]*orb2iner', [-c3*sE, c1*c3*cE, 0]*orb2iner'];

end

function [rot_mat] = rotmax (angle)
% [rot_mat] = rotmax (angle)
%   To obtain the rotation matrix around the X axis given the
%   rotation angle.
% inputs:
%   angle
%       rotation angle, in radians.
% outputs:
%   rot_mat
%       rotation matrix (3, 3)
%

% Valdemir Carrara, Sep, 1998

coan    =  cos(angle);
sian    =  sin(angle);

rot_mat =  [1, 0, 0; 0, coan, sian; 0, -sian, coan];

end

function [rot_mat] = rotmay (angle)
% [rot_mat] = rotmay (angle)
%   To obtain the rotation matrix around the Y axis given the
%   rotation angle.
% inputs:
%   angle
%       rotation angle, in radians.
% outputs:
%   rot_mat
%       rotation matrix (3, 3)
%

% Valdemir Carrara, Sep, 1998


coan    =  cos(angle);
sian    =  sin(angle);

rot_mat =  [coan, 0, -sian; 0, 1, 0; sian, 0, coan];

end

function [rot_mat] = rotmaz (angle)
% [rot_mat] = rotmaz (angle)
%   To obtain the rotation matrix around the Z axis given the
%   rotation angle.
% inputs:
%   angle
%       rotation angle, in radians.
% outputs:
%   rot_mat
%       rotation matrix (3, 3)
%

% Valdemir Carrara, Sep, 1998

coan    =  cos(angle);
sian    =  sin(angle);

rot_mat =  [coan, sian, 0; -sian, coan, 0; 0, 0, 1];
end

function [eccentric] = kepler (mean_anomaly, eccentricity)
% [eccentric] = kepler (mean_anomaly, eccentricity)
%	The subroutine kepler finds a solution to the
%	kepler's equation.
%
% Input:
%	mean_anomaly
%		mean anomaly in radians.
%	eccentricity
%		eccentricity.
%
% Output:
%	eccentric
%		eccentric anomaly in radians.
%
% Authors:
%	Valder M. de Medeiros		june/81		version 2.0
%	Valdemir Carrara			july 2005	(C version)
%   Valdemir Carrara            March/09        Matlab

exc2    = eccentricity*eccentricity;
am1     = mod (mean_anomaly, 2*pi);
am2     = am1 + am1;
am3     = am1 + am2;
shoot   = am1 + eccentricity*(1. - 0.125*exc2)*sin(am1) + ...
		0.5*exc2*(sin(am2) + 0.75*eccentricity*sin(am3));
shoot   = mod (shoot, 2*pi);

e1      = 1.0;
ic      = 0;

while ((abs(e1) > 1.e-12) && (ic <= 10)) 
	e1    = (shoot - am1 - eccentricity*sin(shoot)) / ...
			(1.0 - eccentricity*cos(shoot));
    shoot = shoot - e1;
    ic    = ic + 1;
end

if (ic >= 10)
    disp ('warning ** subroutine kepler did not converge in 10 iterations');
end

eccentric = shoot;


end

== matlab function Thruster_Example_rw/Prac1/Subsystem/RCS_Controller/RCS only attitude and position control ==
  data: p_ref input; u output; p input; v_ref input; v input; q_ref input; q input; w_ref input; w input; RCS_POS input; RCS_DIR input; y_cmd output; y_ach output
function [u, y_cmd, y_ach] = fcn( ...
                                  p_ref, p, v_ref, v, ...          % position control
                                  q_ref, q, w_ref, w, ...          % attitude control (quat + body rates)
                                  RCS_POS, RCS_DIR)                % thruster geometry
%#codegen
% p, v : 3x1 [m], [m/s]
% q_ref, q : 4x1 quaternion (scalar-first: [qw qx qy qz]')
% w_ref, w : 3x1 [rad/s] (body frame)
% RCS_POS : 3xN position vectors of thrusters wrt CoM [m]
% RCS_DIR : 3xN thrust direction unit vectors [N/A] in body frame
% u : Nx1 thrust commands [N]

% ====== Parameters ======
Tmax = 22;       % [N]
m    = 2000;     % [kg]

% Translational PD gains
Kp_p = 2 * diag([1 1 1]);
Kd_p = 4 * diag([1 1 1]);

% Attitude PD gains (원하시면 사용하신 K1,K2 그대로 넣으셔도 됩니다)
Kq = 0.5 * diag([1 1 1]);    % quaternion-vector part gain
Kw = 2  * diag([1 1 1]);    % angular-rate gain

% (선택) 힘/토크 가중치: 단위/스케일 차이 때문에 보통 넣는 걸 권장합니다.
wF   = 1.0;    % force weight
wTau = 1.0;    % torque weight (필요 시 크게/작게 조정)

% ====== 1) Translation: PD -> F_cmd ======
e_p = p_ref - p;
e_v = v_ref - v;

a_cmd = Kp_p*e_p + Kd_p*e_v;
F_cmd = m * a_cmd;              % 3x1

% ====== 2) Attitude: quaternion error + rate error -> Tau_cmd ======
qe = quat_err_scalar_first(q_ref, q);     % q_err = q_ref ⊗ conj(q)
% 쿼터니언 언와인딩 방지(연속성)
if qe(1) < 0
    qe = -qe;
end
qe_v = qe(2:4);

we = w - w_ref;                 % body rate error (원하시면 w_ref-w 로 바꾸셔도 됨)

% 기본적인 PD 토크(부호는 시스템 정의에 맞게 조정 가능)
Tau_cmd = -(Kq*qe_v + Kw*we);    % 3x1

% ====== 3) Build 6xN allocation matrix B ======
N = size(RCS_DIR, 2);

B = zeros(6, N);
for i = 1:N
    ti = RCS_DIR(:, i);          % 3x1
    ri = RCS_POS(:, i);          % 3x1
    B(1:3, i) = ti;
    B(4:6, i) = cross(ri, ti);
end

% ====== 4) Stack command y = [F; Tau] and solve allocation ======
y_cmd = [wF*F_cmd; wTau*Tau_cmd];      % 6x1
Bw    = [wF*B(1:3,:); wTau*B(4:6,:)];  % weighted B

% 간단 대안: pinv + clip + active-set 반복(툴박스 없이 가능)
u = rcs_allocate_pinv_clip_iter(Bw, y_cmd, Tmax);

y_ach = B*u;    % achieved (unweighted, physical)

end

% ===== Helper: iterative clipped pseudo-inverse allocation =====
function u = rcs_allocate_pinv_clip_iter(B, y, Tmax)
%#codegen
N = size(B,2);

% 초기 해
u = pinv(B) * y;

% active-set 반복: 0 또는 Tmax에 걸린 추력기는 고정하고 나머지만 재해결
MAX_IT = 10;
for k = 1:MAX_IT
    u_prev = u;

    % bounds 적용
    u = max(u, 0);
    u = min(u, Tmax);

    % 자유 변수 마스크
    free = (u > 1e-9) & (u < Tmax - 1e-9);

    if ~any(free)
        break;
    end

    % 고정된 변수 기여를 빼고, 자유 변수만 재계산
    y_res = y - B(:, ~free) * u(~free);
    Bf    = B(:, free);

    uf = pinv(Bf) * y_res;

    u(free) = uf;

    % 수렴 체크
    if norm(u - u_prev) < 1e-6
        break;
    end
end
end

% ===== Helper: quaternion error (scalar-first) =====
function qe = quat_err_scalar_first(q_ref, q)
%#codegen
% qe = q_ref ⊗ conj(q)
qc = [q(1); -q(2); -q(3); -q(4)];

qe = quat_mul_scalar_first(q_ref, qc);
end

function q = quat_mul_scalar_first(q1, q2)
%#codegen
w1=q1(1); x1=q1(2); y1=q1(3); z1=q1(4);
w2=q2(1); x2=q2(2); y2=q2(3); z2=q2(4);

q = [ ...
    w1*w2 - x1*x2 - y1*y2 - z1*z2; ...
    w1*x2 + x1*w2 + y1*z2 - z1*y2; ...
    w1*y2 - x1*z2 + y1*w2 + z1*x2; ...
    w1*z2 + x1*y2 - y1*x2 + z1*w2  ...
    ];
end

== matlab function Thruster_Example_rw/Prac1/Subsystem/RCS_Controller/RCS position control ==
  data: p_ref input; out output; p input; v_ref input; v input; RCS_THR_vec input
function out = fcn(p_ref, p, v_ref, v, RCS_THR_vec)
% ====== 파라미터 ======
Tmax   = 22;       % [N]
m = 2000;
% pwmMax = 65535;    % 예: 16-bit
% pwmMin = 0;        % 필요하면 최소 구동값 넣기
Kp = 20*diag([1 1 1]);
Kd = 40*diag([1 1 1]);
% ====== 1) PD -> F_cmd ======
e_p = p_ref - p;
e_v = v_ref - v;

a_cmd = Kp*e_p + Kd*e_v;
F_cmd = m * a_cmd;

% ====== 2) Allocation ======
% [u, F_ach] = rcs_allocate_lsqlin(F_cmd, RCS_THR_vec, Tmax); % toolbox 권장
[u, F_ach] = rcs_allocate_pinv_clip(F_cmd, RCS_THR_vec, Tmax); % 간단 대안

% ====== 3) PWM ======
% pwm = thrust_to_pwm(u, Tmax, pwmMax, pwmMin);
out = u./1;
% (디버그)
% disp("F_cmd  = " + mat2str(F_cmd',4))
% disp("F_ach  = " + mat2str(F_ach',4))
% disp("u(N)   = " + mat2str(u',4))
% disp("pwm    = " + mat2str(pwm',4))

end

function [u, F_ach] = rcs_allocate_pinv_clip(F_cmd, RCS_THR_vec, Tmax)
    B = RCS_THR_vec;     % 3xN
    u = pinv(B) * F_cmd; % unconstrained

    % Thruster는 보통 단방향(0~Tmax)이므로 음수는 0으로
    u = max(u, 0);
    u = min(u, Tmax);

    F_ach = B*u;
end


function pwm = thrust_to_pwm(u, Tmax, pwmMax, pwmMin)
    % u: Nx1 thrust command [N]
    % pwmMax: 예) 65535 또는 255
    % pwmMin: (선택) 밸브/드라이버가 실제로 열리는 최소 duty가 있으면 반영

    duty = u(:) / Tmax;          % 0~1
    duty = max(0, min(1, duty));

    if nargin >= 4 && pwmMin > 0
        % duty>0인 경우에만 최소 구동 듀티 적용(데드존)
        duty(duty>0) = max(duty(duty>0), pwmMin/pwmMax);
    end

    pwm = round(duty * pwmMax);
end

== matlab function Thruster_Example_rw/Prac1/Subsystem/TC Kepler Propagate ==
  data: initial_condition input; dfdt output; F_eci input
function dfdt  = eq_propagate(initial_condition, F_eci)
% Lectures_TwoBodyProblem.pdf
% 우주시스템입문 - 도미타 노부유키 eq(7.8) p136
% https://en.wikipedia.org/wiki/Standard_gravitational_parameter
u  = 3.9860064e+14; % earth gravitional parameter
Re = 6378137;      % earth radius [m]

dfdt = zeros(size(initial_condition));

% x=x
% x1=dx/dt
% dx1/dt = d^2(x)/dt

x1 = initial_condition(4); % x1 = dx/dt
y1 = initial_condition(5); % y1 = dy/dt
z1 = initial_condition(6); % z1 = dz/dt
x  = initial_condition(1); % x
y  = initial_condition(2); % y
z  = initial_condition(3); % z

r=sqrt(x^2+y^2+z^2);

% % %   Keplar Motion Equatnion
% % %  => r_dd + u/(r^3)r_ = 0 => r_dd = -u/(r^3)r_
dfdt(1) = x1;
dfdt(2) = y1;
dfdt(3) = z1;
dfdt(4) = -u*x/(r^3) + F_eci(1);
dfdt(5) = -u*y/(r^3) + F_eci(2);
dfdt(6) = -u*z/(r^3) + F_eci(3);

end

== matlab function Thruster_Example_rw/Prac1/Subsystem/THR_Allocation ==
  data: pwm output; tau_cmd input; F_on input; f input; r_thr input
function pwm = RCS_Torque2PWM(tau_cmd, F_on, f, r_thr)
%#codegen
% ============================================================
% Minimal RCS allocation: torque command -> PWM duty (0..1)
%   tau ≈ sum_i r_i x (f_i * F_on_i * pwm_i)
%
% Inputs:
%   tau_cmd [3x1]
%   F_on    scalar or [12x1]
%   f       [3x12]  (columns are unit vectors)
%   r_thr   [3x12]  (columns are position vectors wrt CoM)
%
% Output:
%   pwm     [12x1] duty in [0,1]
% ============================================================
N = 16;
% F_on -> 12x1
if isscalar(F_on)
    Fon = F_on * ones(N,1);
else
    Fon = F_on(:);
end

% Build effectiveness matrix B (3x12): tau = B * pwm
B = zeros(3,N);
for i = 1:N
    Fi = Fon(i);
    B(:,i) = cross3(r_thr(:,i), f(:,i) * Fi);  % torque from pwm=1
end

% Unconstrained least-squares solution (minimum-norm)
pwm = B' * ((B*B') \ tau_cmd);

% Clamp to [0,1]
for i=1:N
    if pwm(i) < 0, pwm(i) = 0; end
    if pwm(i) > 1, pwm(i) = 1; end
end

end

function c = cross3(a,b)
c = [ a(2)*b(3) - a(3)*b(2);
      a(3)*b(1) - a(1)*b(3);
      a(1)*b(2) - a(2)*b(1) ];
end
